simulink subsystem "ApplAbFOCSL"  (R2024b)
settings: Solver=VariableStepAuto  StartTime=0.0  StopTime=10.0  RelTol=1e-3
settings Model: Creator=The MathWorks, Inc.  LastModifiedBy=The MathWorks, Inc.
settings RTWCC: GPUComputeCapability=3.5

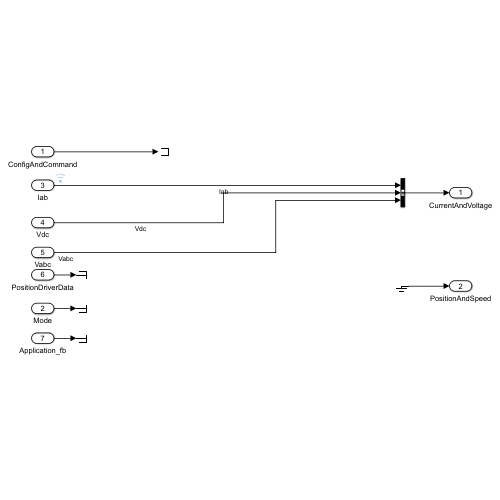
[thumbnail: Simulink's stored preview of the top-level diagram]
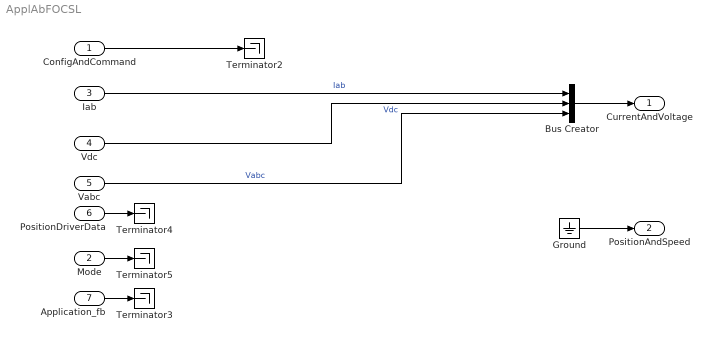
== system ApplAbFOCSL ==
  ConfigAndCommand : Inport
  Mode : Inport  Port=2
  Iab : Inport  Port=3
  Vdc : Inport  Port=4
  Vabc : Inport  Port=5
  PositionDriverData : Inport  Port=6
  Application_fb : Inport  Port=7
  Bus Creator : BusCreator  Inputs=3
  Ground : Ground
  Terminator{2..5} (4 alike) : Terminator
  CurrentAndVoltage : Outport
  PositionAndSpeed : Outport  Port=2
  wires:
  Vdc/1 -> Bus Creator/2  "Vdc"
  Bus Creator/1 -> CurrentAndVoltage/1
  Iab/1 -> Bus Creator/1  "Iab"
  ConfigAndCommand/1 -> Terminator2/1
  Application_fb/1 -> Terminator3/1
  PositionDriverData/1 -> Terminator4/1
  Mode/1 -> Terminator5/1
  Ground/1 -> PositionAndSpeed/1
  Vabc/1 -> Bus Creator/3  "Vabc"
